simulink model "EMPEL_Project_Final"  (R2024a)
settings: Solver=ode4  StartTime=0.0  StopTime=0.15  FixedStep=Ts  RelTol=1e-3
undefined symbols (not defined in the file): Ts
libraries: spsMeanLib x6, spsCurrentMeasurementLib x4, spsSeriesRLCBranchLib x3, spsVoltageMeasurementLib x3, spsDCVoltageSourceLib x1, spsDiodeLib x1, spsGroundLib x1, spsMosfetLib x1, spsPWMGeneratorDCDCLib x1, sps_lib x1
settings Model: Creator=Rucha  LastModifiedBy=Rucha

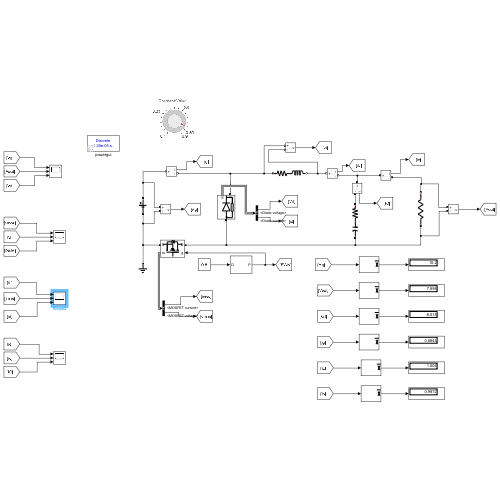
[thumbnail: Simulink's stored preview of the top-level diagram]
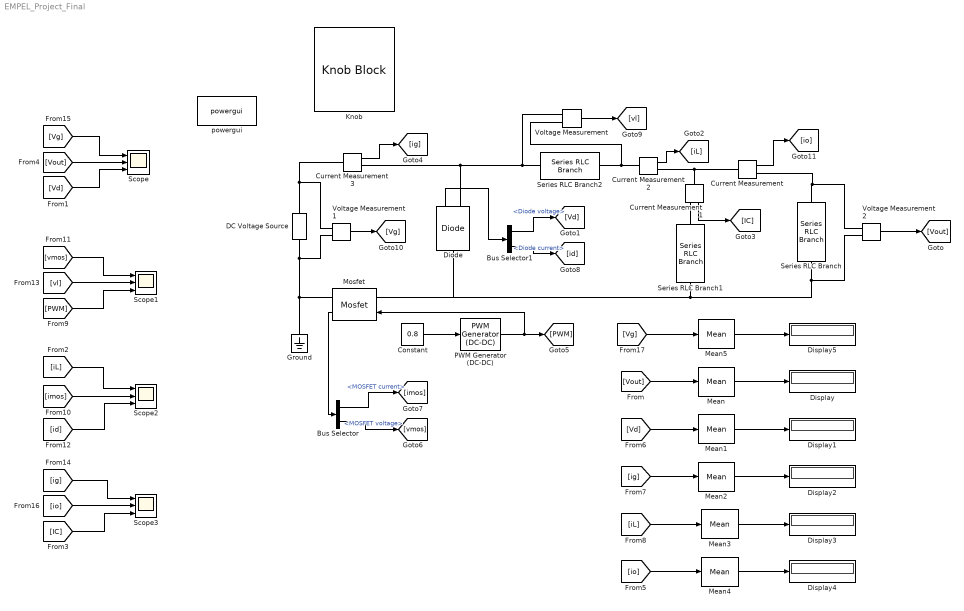
== system EMPEL_Project_Final ==
  Bus Selector : BusSelector  OutputSignals=MOSFET current,MOSFET voltage
  Bus Selector1 : BusSelector  OutputSignals=Diode voltage,Diode current
  Constant : Constant  Value=0.8
  Current Measurement{,1..3} (4 alike) : spsCurrentMeasurementLib/Current Measurement  PhasorSimulation=off  OutputType=Complex  PSBequivalent=0
  DC Voltage Source : spsDCVoltageSourceLib/DC Voltage Source  Amplitude=10.2  Measurements=None
  Diode : spsDiodeLib/Diode  Ron=0.4  Lon=0  Vf=1.0  IC=0  UseSnubber=0  Rs=1e6  Cs=1e6  Measurements=on
  Display{,1..5} (6 alike) : Display
  Ground : spsGroundLib/Ground  LConnTagsString=a
  Knob : KnobBlock  ScaleMin=0.1  ScaleMax=0.9  TickInterval=0.25
  Mean{,1..5} (6 alike) : spsMeanLib/Mean  Freq=fsw  Vinit=0  Ts=Ts
  Mosfet : spsMosfetLib/Mosfet  Ron=17.5e-3  Lon=0  Rd=1e-10  Vfd=1.3  IC=0  Rs=inf  Cs=0  Measurements=on
  PWM Generator (DC-DC) : spsPWMGeneratorDCDCLib/PWM Generator (DC-DC)  Fsw=fsw  Ts=Ts
  Scope{,1..3} (4 alike) : Scope  NumInputPorts=3
  Series RLC Branch : spsSeriesRLCBranchLib/Series RLC Branch  LConnTagsString=__new0  RConnTagsString=__new0  BranchType=R  Resistance=8  Inductance=1e-3  SetiL0=off  InitialCurrent=0  Capacitance=1e-6  Setx0=off  InitialVoltage=0  Measurements=None
  Series RLC Branch1 : spsSeriesRLCBranchLib/Series RLC Branch  LConnTagsString=__new0  RConnTagsString=__new0  BranchType=RC  Resistance=0.1  Inductance=1e-3  SetiL0=off  InitialCurrent=0  Capacitance=220e-6  Setx0=off  InitialVoltage=0  Measurements=None
  Series RLC Branch2 : spsSeriesRLCBranchLib/Series RLC Branch  LConnTagsString=__new0  RConnTagsString=__new0  BranchType=RL  Resistance=0.6  Inductance=1e-3  SetiL0=off  InitialCurrent=0  Capacitance=1e-6  Setx0=off  InitialVoltage=0  Measurements=None
  Voltage Measurement : spsVoltageMeasurementLib/Voltage Measurement  PhasorSimulation=off  OutputType=Complex  PSBequivalent=0
  Voltage Measurement1 : spsVoltageMeasurementLib/Voltage Measurement  PhasorSimulation=off  OutputType=Complex  PSBequivalent=0
  Voltage Measurement2 : spsVoltageMeasurementLib/Voltage Measurement  PhasorSimulation=off  OutputType=Complex  PSBequivalent=0
  powergui : sps_lib/powergui  Priority=1  SimulationMode=Discrete  SampleTime=Ts  frequency=60  Iterations=50  frequencyindice=0  Pbase=100e6  ErrMax=1e-4  UnitsV=kV  UnitsW=MW  buscounter=0  FunctionMessages=off  echomessages=off  EnableUseOfTLC=off  CurrentSourceSwitches=off  DisableSnubberDevices=off  DisableRonSwitches=off  DisableVfSwitches=off  DisplayEquations=off  AutomaticDiscreteSolvers=off  SolverType=Tustin/Backward Euler (TBE)  Interpol=off  ExternalGateDelay=off  methode=off  Ts=100  x0status=blocks  SPID=on  SwTol=0  HookPort=off  NonlinearTolerance=1e-4  nMaxIteration=100  ContinueOnMaxIteration=off  RestoreLinks=warning  ResistiveCurrentMeasurement=off  Frange=[0:2:500]  Ylog=off  Xlog=on  ShowGrid=off  save=off  variable=ZData  structure=0  ZoomFFT=off  StartTime=0.0  cycles=1  DisplayStyle=1  fundamental=60  FreqAxis=off  MaxFrequency=1000  frequencyindicesteady=1  RmsSteady=1  display=off
  wires:
  Voltage Measurement2/1 -> [Vout]
  Current Measurement2/1 -> [iL]
  Current Measurement1/1 -> [IC]
  [Vout] -> Mean/1
  Mean/1 -> Display/1
  [Vd] -> Mean1/1
  Mean1/1 -> Display1/1
  Current Measurement3/1 -> [ig]
  Mean2/1 -> Display2/1
  [ig] -> Mean2/1
  [iL] -> Mean3/1
  Mean3/1 -> Display3/1
  PWM Generator (DC-DC)/1 -> [PWM], Mosfet/1
  Constant/1 -> PWM Generator (DC-DC)/1
  Mosfet/1 -> Bus Selector/1
  Bus Selector/1 -> [imos]  "<MOSFET current>"
  Bus Selector/2 -> [vmos]  "<MOSFET voltage>"
  Diode/1 -> Bus Selector1/1
  Bus Selector1/1 -> [Vd]  "<Diode voltage>"
  Bus Selector1/2 -> [id]  "<Diode current>"
  Voltage Measurement/1 -> [vl]
  Voltage Measurement1/1 -> [Vg]
  Current Measurement/1 -> [io]
  [Vg] -> Scope/1
  [Vout] -> Scope/2
  [Vd] -> Scope/3
  [vmos] -> Scope1/1
  [vl] -> Scope1/2
  [PWM] -> Scope1/3
  [imos] -> Scope2/2
  [iL] -> Scope2/1
  [ig] -> Scope3/1
  [io] -> Scope3/2
  [id] -> Scope2/3
  [IC] -> Scope3/3
  [io] -> Mean4/1
  Mean4/1 -> Display4/1
  [Vg] -> Mean5/1
  Mean5/1 -> Display5/1
  connections:
  Current Measurement1/RConn1 -- Series RLC Branch1/LConn1
  Series RLC Branch/RConn1 -- Voltage Measurement2/LConn2 -- Diode/LConn1 -- Mosfet/LConn1 -- Series RLC Branch1/RConn1
  Series RLC Branch2/RConn1 -- Voltage Measurement/LConn2 -- Current Measurement2/LConn1
  Voltage Measurement2/LConn1 -- Current Measurement/RConn1 -- Series RLC Branch/LConn1
  DC Voltage Source/RConn1 -- Voltage Measurement1/LConn1 -- Current Measurement3/LConn1
  Series RLC Branch2/LConn1 -- Diode/RConn1 -- Current Measurement3/RConn1 -- Voltage Measurement/LConn1
  DC Voltage Source/LConn1 -- Ground/LConn1 -- Mosfet/RConn1 -- Voltage Measurement1/LConn2
  Current Measurement1/LConn1 -- Current Measurement/LConn1 -- Current Measurement2/RConn1
